simulink model "Day3_1_1"  (R2022b)
settings: Solver=VariableStepAuto  StartTime=0.0  StopTime=10.0  RelTol=1e-3
values from neighbouring files (symbols this model uses):
  control_gain = 1    [Day3_1.m]
  cs = 1000    [Day3_1.m]
  ks = 30000    [Day3_1.m]
  kt = 300000    [Day3_1.m]
  ms = 500    [Day3_1.m]
  mus = 25    [Day3_1.m]
settings Model: Creator=user  LastModifiedBy=user

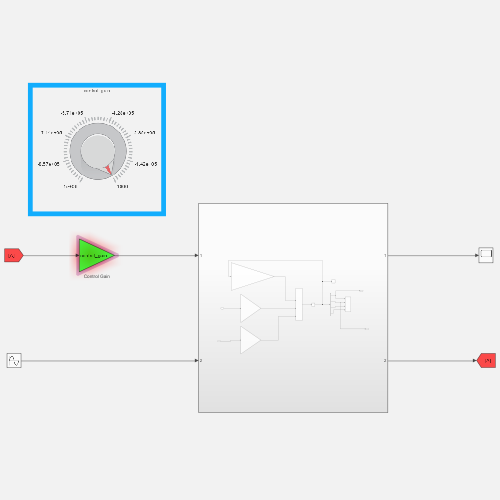
[thumbnail: Simulink's stored preview of the top-level diagram]
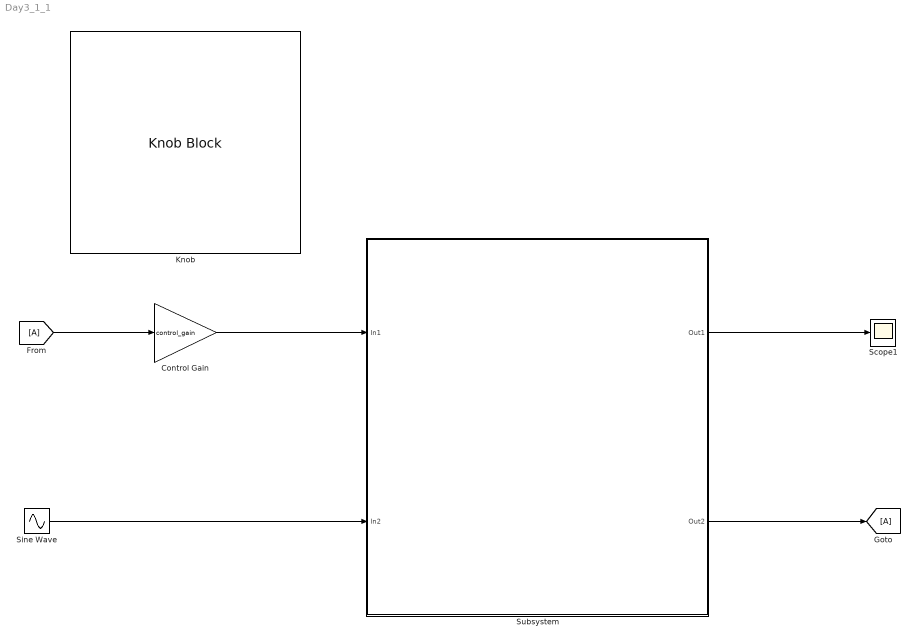
== system Day3_1_1 ==
  Control Gain : Gain  Gain=control_gain
  From : From
  Goto : Goto
  Knob : KnobBlock  ScaleMin=-1000000  ScaleMax=1000
  Scope1 : Scope
  Sine Wave : Sin  SampleTime=0
  Subsystem : Subsystem
  wires:
  Subsystem/2(Out2) -> Goto/1
  From/1 -> Control Gain/1
  Subsystem/1(Out1) -> Scope1/1
  Control Gain/1 -> Subsystem/1(In1)
  Sine Wave/1 -> Subsystem/2(In2)

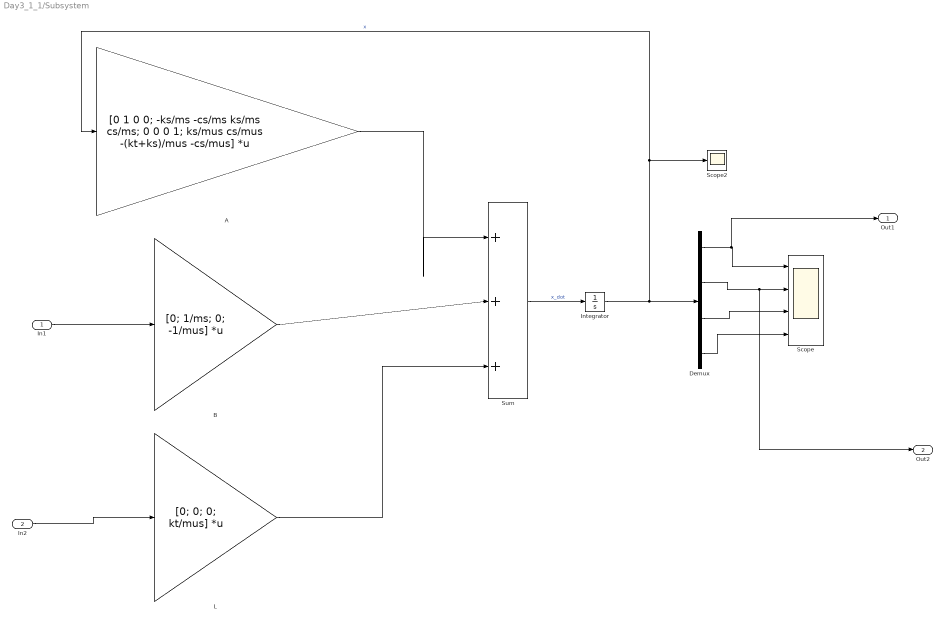
== system Day3_1_1/Subsystem ==
  In1 : Inport
  In2 : Inport  Port=2
  A : Gain  Gain=[0 1 0 0; -ks/ms -cs/ms ks/ms cs/ms; 0 0 0 1; ks/mus cs/mus -(kt+ks)/mus -cs/mus]  Multiplication=Matrix(K*u)
  B : Gain  Gain=[0; 1/ms; 0; -1/mus]  Multiplication=Matrix(K*u)
  Demux : Demux
  Integrator : Integrator
  L : Gain  Gain=[0; 0; 0; kt/mus]  Multiplication=Matrix(K*u)
  Scope : Scope  NumInputPorts=4
  Scope2 : Scope
  Sum : Sum  Inputs=|+++
  Out1 : Outport
  Out2 : Outport  Port=2
  wires:
  Demux/1 -> Out1/1, Scope/1
  A/1 -> Sum/1
  Integrator/1 -> Demux/1, A/1, Scope2/1  "x"
  L/1 -> Sum/3
  B/1 -> Sum/2
  Demux/3 -> Scope/3
  Sum/1 -> Integrator/1  "x_dot"
  In1/1 -> B/1
  Demux/4 -> Scope/4
  Demux/2 -> Out2/1, Scope/2
  In2/1 -> L/1
